simulink library "Div_by_0_protection"  (R2018b)
settings: Solver=VariableStepAuto  StartTime=0.0  StopTime=10.0  RelTol=1e-3
undefined symbols (not defined in the file or in its folder): fswParams
libraries: two_norm x1
settings Model: Creator=colem  LastModifiedBy=colem

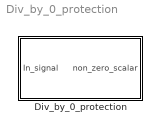
== system Div_by_0_protection ==
  Div_by_0_protection : Subsystem

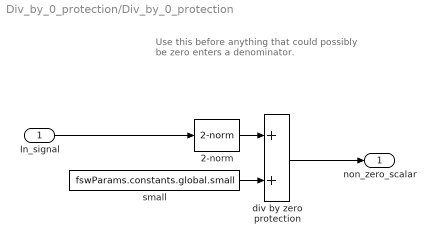
== system Div_by_0_protection/Div_by_0_protection ==
  note: Use this before anything that could possibly be zero enters a denominator.
  In_signal : Inport
  2-norm : two_norm/2-norm  SystemSampleTime=-1
  div by zero protection : Sum
  small : Constant  Value=fswParams.constants.global.small  SampleTime=fswParams.sample_time_s
  non_zero_scalar : Outport
  wires:
  2-norm/1 -> div by zero protection/1
  small/1 -> div by zero protection/2
  div by zero protection/1 -> non_zero_scalar/1
  In_signal/1 -> 2-norm/1
